simulink model "ques1"  (R2021a)
settings: Solver=VariableStepAuto  StartTime=0.0  StopTime=10.0  RelTol=1e-3
model workspace (MAT data in the model file):
  b = Simulink.Parameter
  b.Value = 50
  b.DataType = 'auto'
  b.Dimensions = [1 1]
  k1 = Simulink.Parameter
  k1.Value = 50
  k1.DataType = 'auto'
  k1.Dimensions = [1 1]
  k12 = Simulink.Parameter
  k12.Value = 1000
  k12.DataType = 'auto'
  k12.Dimensions = [1 1]
  m1 = Simulink.Parameter
  m1.Value = 100
  m1.DataType = 'auto'
  m1.Dimensions = [1 1]
  m2 = Simulink.Parameter
  m2.Value = 100
  m2.DataType = 'auto'
  m2.Dimensions = [1 1]
settings Model: OrderedModelArguments=off  Creator=AVM  LastModifiedBy=AVM

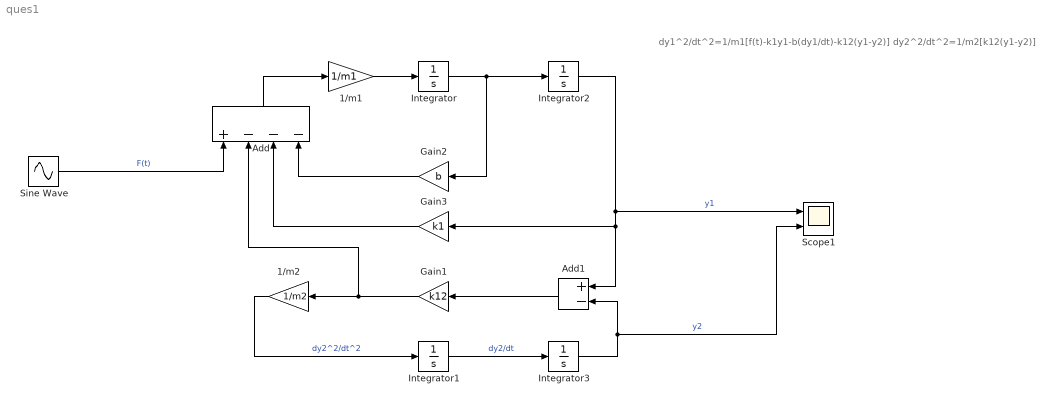
== system ques1 ==
  note: dy1^2/dt^2=1/m1[f(t)-k1y1-b(dy1/dt)-k12(y1-y2)]
      | dy2^2/dt^2=1/m2[k12(y1-y2)]
  1/m1 : Gain  Gain=1/m1
  1/m2 : Gain  Gain=1/m2
  Add : Sum  Inputs=+---
  Add1 : Sum  Inputs=+-
  Gain1 : Gain  Gain=k12
  Gain2 : Gain  Gain=b
  Gain3 : Gain  Gain=k1
  Integrator{,1..3} (4 alike) : Integrator
  Scope1 : Scope  NumInputPorts=2
  Sine Wave : Sin  Amplitude=2  Frequency=10  SampleTime=0
  wires:
  Integrator/1 -> Gain2/1, Integrator2/1
  Gain2/1 -> Add/4
  Integrator1/1 -> Integrator3/1  "dy2/dt"
  Gain3/1 -> Add/3
  Gain1/1 -> Add/2, 1/m2/1
  Integrator3/1 -> Scope1/2, Add1/2  "y2"
  1/m1/1 -> Integrator/1
  1/m2/1 -> Integrator1/1  "dy2^2/dt^2"
  Add1/1 -> Gain1/1
  Integrator2/1 -> Gain3/1, Add1/1, Scope1/1  "y1"
  Add/1 -> 1/m1/1
  Sine Wave/1 -> Add/1  "F(t)"
